simulink model "Pt_Diff_CS803"  (Simulink 7.0)
settings: Solver=ode45  StartTime=0  StopTime=20  FixedStep=TSTEP  RelTol=1e-3
PreLoadFcn:
  | cd extensions\simulink\pt_diff
  | Run_ft4wd_eclass
  | lsd_parameta_eclass
  | cd ..\..\..
undefined symbols (not defined in the file): LOCKED_FD_DAMP, LOCKED_FD_K, LOCKED_FD_OPT, LOCKED_RD_DAMP, LOCKED_RD_K, LOCKED_RD_OPT, LOCKED_XC_DAMP, LOCKED_XC_K, LOCKED_XC_OPT, M_DIFF_FD_TABLE, M_DIFF_RD_TABLE, M_DIFF_XC_TABLE, R_EFF_F_FD, R_EFF_F_RD, R_EFF_F_XC, R_EFF_R_FD, R_EFF_R_RD, R_EFF_R_XC, R_GEAR_FD, R_GEAR_RD, R_GEAR_XC, R_REAR_XC
libraries: Solver_SF x1
settings Model: Creator=dhall  LastModifiedBy=ywata  ExtModeTrigMode=oneshot  ExtModeArmWhenConnect=off
settings DataIOCC: LimitDataPoints=off  SaveOutput=off  SaveTime=off  SignalLoggingName=sigsOut
settings OptimizationCC: BooleanDataType=off
settings DebuggingCC: SaveWithParameterizedLinksMsg=none  SignalResolutionControl=TryResolveAllWithWarning  SolverPrmCheckMsg=none  MultiTaskDSMMsg=warning  MultiTaskCondExecSysMsg=none  StrictBusMsg=None
settings HardwareCC: TargetUnknown=on
settings RTWCC: IncludeERTFirstTime=on
settings GRTTargetCC: TargetFcnLib=ansi_tfl_tmw.mat  ModelReferenceCompliant=off  MatFileLogging=off

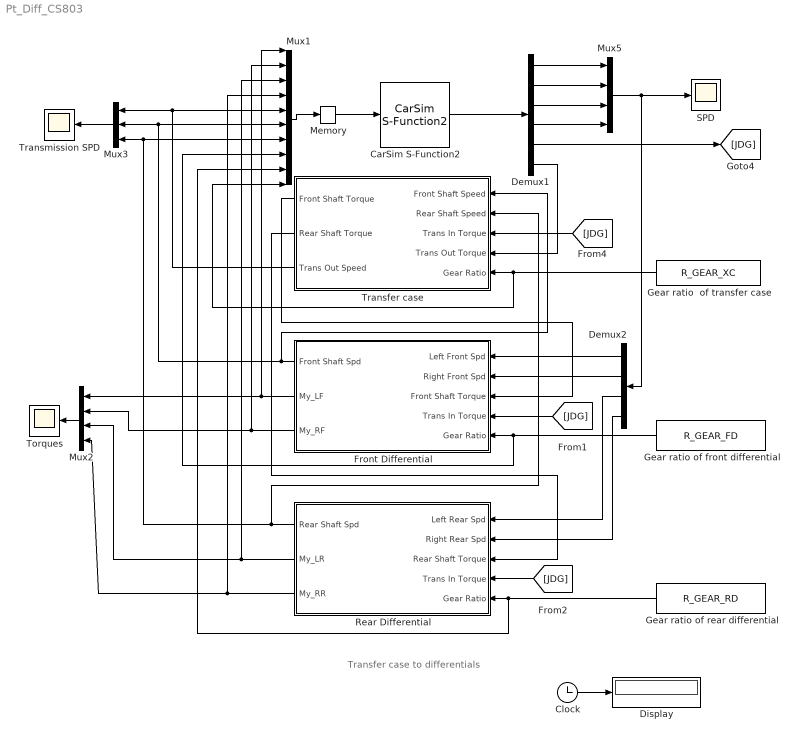
== system Pt_Diff_CS803 ==
  note: Transfer case to differentials
  CarSim S-Function2 : Solver_SF/CarSim S-Function2  Priority=1  VehicleCode=???
      settings: AttributesFormatString=Vehicle Code: %<VehicleCode>
  Clock : Clock
      settings: Decimation=10
  Demux1 : Demux  Outputs=6
  Demux2 : Demux  Orientation=left
  Display : Display
  "Front Differential " : Subsystem  Orientation=left
  Gear ratio  of transfer case : Constant  Orientation=left  Value=R_GEAR_XC  OutDataType=sfix(16)  OutScaling=2^0
  Gear ratio of front differential : Constant  Orientation=left  Value=R_GEAR_FD  OutDataType=sfix(16)  OutScaling=2^0
  Gear ratio of rear differential : Constant  Orientation=left  Value=R_GEAR_RD  OutDataType=sfix(16)  OutScaling=2^0
  Memory : Memory
  Mux1 : Mux  Inputs=10
  Mux2 : Mux  Orientation=left
  Mux3 : Mux  Orientation=left  Inputs=3
  Mux5 : Mux
  Rear Differential : Subsystem  Orientation=left
  SPD : Scope
      settings: YMin=-68.0473  YMax=1340.24
  Torques : Scope
      settings: YMin=0  YMax=1750
  Transfer case : Subsystem  Orientation=left
  Transmission SPD : Scope
      settings: YMin=-111.446  YMax=3683.73
  wires:
  Mux2/1 -> Torques/1
  "Front Differential "/1(Front Shaft Spd) -> Transfer case/1(Front Shaft Speed), Mux1/6, Mux3/2
  Rear Differential/1(Rear Shaft Spd) -> Transfer case/2(Rear Shaft Speed), Mux1/7, Mux3/3
  Transfer case/1(Front Shaft Torque) -> "Front Differential "/3(Front Shaft Torque)
  Transfer case/2(Rear Shaft Torque) -> Rear Differential/3(Rear Shaft Torque)
  [JDG] -> Rear Differential/4(Trans In Torque)
  [JDG] -> Transfer case/3(Trans In Torque)
  Mux5/1 -> SPD/1, Demux2/1
  Demux2/1 -> "Front Differential "/1(Left Front Spd)
  Demux2/2 -> "Front Differential "/2(Right Front Spd)
  Demux2/3 -> Rear Differential/1(Left Rear Spd)
  Demux2/4 -> Rear Differential/2(Right Rear Spd)
  [JDG] -> "Front Differential "/4(Trans In Torque)
  Mux1/1 -> Memory/1
  "Front Differential "/2(My_LF) -> Mux1/1, Mux2/1
  "Front Differential "/3(My_RF) -> Mux1/2, Mux2/2
  Rear Differential/2(My_LR) -> Mux1/3, Mux2/3
  Rear Differential/3(My_RR) -> Mux1/4, Mux2/4
  Gear ratio of rear differential/1 -> Rear Differential/5(Gear Ratio), Mux1/9
  Gear ratio of front differential/1 -> "Front Differential "/5(Gear Ratio), Mux1/8
  Gear ratio  of transfer case/1 -> Transfer case/5(Gear Ratio), Mux1/10
  Transfer case/3(Trans Out Speed) -> Mux1/5, Mux3/1
  Clock/1 -> Display/1
  CarSim S-Function2/1 -> Demux1/1
  Memory/1 -> CarSim S-Function2/1
  Mux3/1 -> Transmission SPD/1
  Demux1/1 -> Mux5/1
  Demux1/2 -> Mux5/2
  Demux1/3 -> Mux5/3
  Demux1/4 -> Mux5/4
  Demux1/5 -> [JDG]
  Demux1/6 -> Transfer case/4(Trans Out Torque)

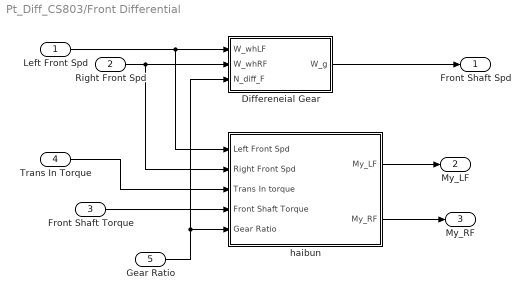
== system Pt_Diff_CS803/Front Differential  ==
  Left Front Spd : Inport  OutDataType=sfix(16)  OutScaling=2^0
  Right Front Spd : Inport  Port=2  OutDataType=sfix(16)  OutScaling=2^0
  Front Shaft Torque : Inport  Port=3  OutDataType=sfix(16)  OutScaling=2^0
  Trans In Torque : Inport  Port=4  OutDataType=sfix(16)  OutScaling=2^0
  Gear Ratio : Inport  Port=5  OutDataType=sfix(16)  OutScaling=2^0
  Differeneial Gear : Subsystem
  haibun : Subsystem
  Front Shaft Spd : Outport
  My_LF : Outport  Port=2
  My_RF : Outport  Port=3
  wires:
  haibun/2(My_RF) -> My_RF/1
  haibun/1(My_LF) -> My_LF/1
  Right Front Spd/1 -> Differeneial Gear/2(W_whRF), haibun/2(Right Front Spd)
  Left Front Spd/1 -> Differeneial Gear/1(W_whLF), haibun/1(Left Front Spd)
  Gear Ratio/1 -> haibun/5(Gear Ratio), Differeneial Gear/3(N_diff_F)
  Differeneial Gear/1(W_g) -> Front Shaft Spd/1
  Front Shaft Torque/1 -> haibun/4(Front Shaft Torque)
  Trans In Torque/1 -> haibun/3(Trans In torque)

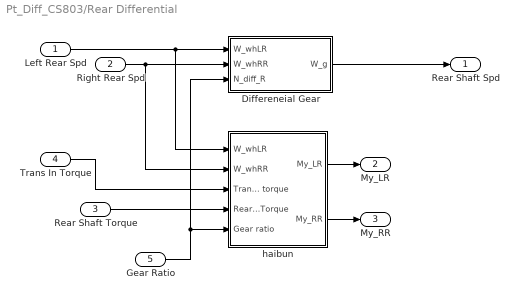
== system Pt_Diff_CS803/Rear Differential ==
  Left Rear Spd : Inport  OutDataType=sfix(16)  OutScaling=2^0
  Right Rear Spd : Inport  Port=2  OutDataType=sfix(16)  OutScaling=2^0
  Rear Shaft Torque : Inport  Port=3  OutDataType=sfix(16)  OutScaling=2^0
  Trans In Torque : Inport  Port=4  OutDataType=sfix(16)  OutScaling=2^0
  Gear Ratio : Inport  Port=5  OutDataType=sfix(16)  OutScaling=2^0
  Differeneial Gear : Subsystem
  haibun : Subsystem
  Rear Shaft Spd : Outport
  My_LR : Outport  Port=2
  My_RR : Outport  Port=3
  wires:
  Trans In Torque/1 -> haibun/3(Trans In torque)
  Rear Shaft Torque/1 -> haibun/4(Rear Shaft Torque)
  Differeneial Gear/1(W_g) -> Rear Shaft Spd/1
  Gear Ratio/1 -> Differeneial Gear/3(N_diff_R), haibun/5(Gear ratio)
  Left Rear Spd/1 -> haibun/1(W_whLR), Differeneial Gear/1(W_whLR)
  Right Rear Spd/1 -> haibun/2(W_whRR), Differeneial Gear/2(W_whRR)
  haibun/1(My_LR) -> My_LR/1
  haibun/2(My_RR) -> My_RR/1

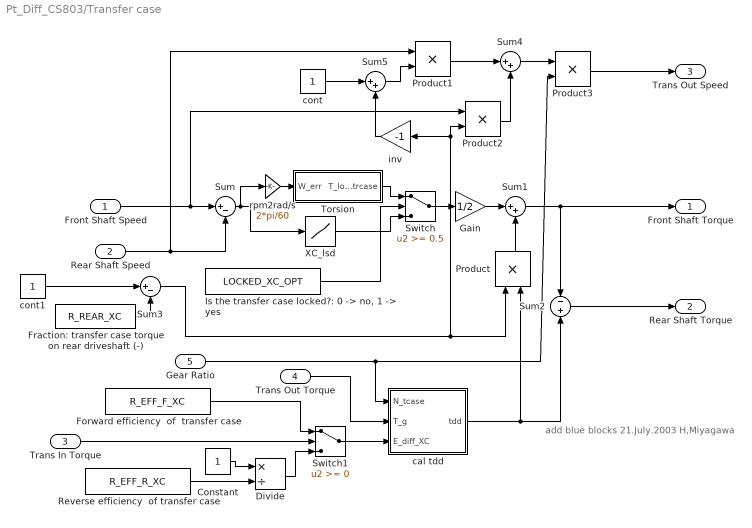
== system Pt_Diff_CS803/Transfer case ==
  note: add blue blocks
      | 21.July.2003
      | H,Miyagawa
  Front Shaft Speed : Inport  OutDataType=sfix(16)  OutScaling=2^0
  Rear Shaft Speed : Inport  Port=2  OutDataType=sfix(16)  OutScaling=2^0
  Trans In Torque : Inport  Port=3  OutDataType=sfix(16)  OutScaling=2^0
  Trans Out Torque : Inport  Port=4  OutDataType=sfix(16)  OutScaling=2^0
  Gear Ratio : Inport  Port=5  OutDataType=sfix(16)  OutScaling=2^0
  Constant : Constant  OutDataType=sfix(16)  OutScaling=2^0
  Divide : Product  Inputs=*/  OutDataType=sfix(16)  OutScaling=2^0  InputSameDT=on
  Forward efficiency  of  transfer case : Constant  Value=R_EFF_F_XC  OutDataType=sfix(16)  OutScaling=2^0
  Fraction: transfer case torque on rear driveshaft (-) : Constant  Value=R_REAR_XC  OutDataType=sfix(16)  OutScaling=2^0
  Gain : Gain  Gain=1/2  ParameterDataType=sfix(16)  ParameterScaling=2^0  OutDataType=sfix(16)  OutScaling=2^0  SaturateOnIntegerOverflow=on
  "Is the transfer case locked?: 0 -> no, 1 -> yes" : Constant  Value=LOCKED_XC_OPT  OutDataType=sfix(16)  OutScaling=2^0
  Product : Product  Orientation=up  OutDataType=sfix(16)  OutScaling=2^0  SaturateOnIntegerOverflow=on  InputSameDT=on
  Product1 : Product  OutDataType=sfix(16)  OutScaling=2^0  SaturateOnIntegerOverflow=on  InputSameDT=on
  Product2 : Product  OutDataType=sfix(16)  OutScaling=2^0  SaturateOnIntegerOverflow=on  InputSameDT=on
  Product3 : Product  OutDataType=sfix(16)  OutScaling=2^0  SaturateOnIntegerOverflow=on  InputSameDT=on
  Reverse efficiency  of transfer case : Constant  Value=R_EFF_R_XC  OutDataType=sfix(16)  OutScaling=2^0
  Sum : Sum  Inputs=|+-  OutDataType=sfix(16)  OutScaling=2^0  SaturateOnIntegerOverflow=on  InputSameDT=on
  Sum1 : Sum  Inputs=|++  OutDataType=sfix(16)  OutScaling=2^0  SaturateOnIntegerOverflow=on  InputSameDT=on
  Sum2 : Sum  Inputs=-|+  OutDataType=sfix(16)  OutScaling=2^0  SaturateOnIntegerOverflow=on  InputSameDT=on
  Sum3 : Sum  Inputs=|+-  OutDataType=sfix(16)  OutScaling=2^0  SaturateOnIntegerOverflow=on  InputSameDT=on
  Sum4 : Sum  Inputs=|++  OutDataType=sfix(16)  OutScaling=2^0  SaturateOnIntegerOverflow=on  InputSameDT=on
  Sum5 : Sum  Inputs=|++  OutDataType=sfix(16)  OutScaling=2^0  SaturateOnIntegerOverflow=on  InputSameDT=on
  Switch : Switch  Threshold=0.5  SaturateOnIntegerOverflow=on  InputSameDT=on
  Switch1 : Switch  SaturateOnIntegerOverflow=on  InputSameDT=on
  Torsion : Subsystem
  XC_lsd : Lookup  InputValues=M_DIFF_XC_TABLE(:,1)  Table=M_DIFF_XC_TABLE(:,2)  OutDataType=sfix(16)  OutScaling=2^0  SaturateOnIntegerOverflow=on
  cal tdd : Subsystem
  cont : Constant  OutDataType=sfix(16)  OutScaling=2^0
  cont1 : Constant  OutDataType=sfix(16)  OutScaling=2^0
  inv : Gain  Orientation=left  Gain=-1  ParameterDataType=sfix(16)  ParameterScaling=2^0  OutDataType=sfix(16)  OutScaling=2^0  SaturateOnIntegerOverflow=on
  rpm2rad/s : Gain  Gain=2*pi/60  ParameterDataType=sfix(16)  ParameterScaling=2^0  OutDataType=sfix(16)  OutScaling=2^0  SaturateOnIntegerOverflow=on
  Front Shaft Torque : Outport
  Rear Shaft Torque : Outport  Port=2
  Trans Out Speed : Outport  Port=3
  wires:
  Sum1/1 -> Sum2/1, Front Shaft Torque/1
  Sum2/1 -> Rear Shaft Torque/1
  cal tdd/1(tdd) -> Product/2, Sum2/2
  Switch1/1 -> cal tdd/3(E_diff_XC)
  Forward efficiency  of  transfer case/1 -> Switch1/1
  Trans In Torque/1 -> Switch1/2
  Trans Out Torque/1 -> cal tdd/2(T_g)
  Product/1 -> Sum1/2
  Gain/1 -> Sum1/1
  Switch/1 -> Gain/1
  XC_lsd/1 -> Switch/3
  "Is the transfer case locked?: 0 -> no, 1 -> yes"/1 -> Switch/2
  Sum/1 -> XC_lsd/1, rpm2rad/s/1
  Torsion/1(T_lock_trcase) -> Switch/1
  Product2/1 -> Sum4/2
  Product1/1 -> Sum4/1
  Sum4/1 -> Product3/1
  Product3/1 -> Trans Out Speed/1
  Gear Ratio/1 -> cal tdd/1(N_tcase), Product3/2
  Sum5/1 -> Product1/2
  cont/1 -> Sum5/1
  inv/1 -> Sum5/2
  Front Shaft Speed/1 -> Sum/1, Product2/1
  Rear Shaft Speed/1 -> Sum/2, Product1/1
  Fraction: transfer case torque on rear driveshaft (-)/1 -> Sum3/2
  Sum3/1 -> Product/1, Product2/2, inv/1
  cont1/1 -> Sum3/1
  Constant/1 -> Divide/1
  Reverse efficiency  of transfer case/1 -> Divide/2
  Divide/1 -> Switch1/3
  rpm2rad/s/1 -> Torsion/1(W_err)

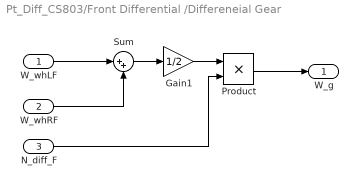
== system Pt_Diff_CS803/Front Differential /Differeneial Gear ==
  W_whLF : Inport  OutDataType=sfix(16)  OutScaling=2^0
  W_whRF : Inport  Port=2  OutDataType=sfix(16)  OutScaling=2^0
  N_diff_F : Inport  Port=3  OutDataType=sfix(16)  OutScaling=2^0
  Gain1 : Gain  Gain=1/2  ParameterDataType=sfix(16)  ParameterScaling=2^0  OutDataType=sfix(16)  OutScaling=2^0  SaturateOnIntegerOverflow=on
  Product : Product  OutDataType=sfix(16)  OutScaling=2^0  SaturateOnIntegerOverflow=on  InputSameDT=on
  Sum : Sum  Inputs=|++  OutDataType=sfix(16)  OutScaling=2^0  SaturateOnIntegerOverflow=on  InputSameDT=on
  W_g : Outport
  wires:
  Product/1 -> W_g/1
  Gain1/1 -> Product/1
  W_whRF/1 -> Sum/2
  W_whLF/1 -> Sum/1
  N_diff_F/1 -> Product/2
  Sum/1 -> Gain1/1

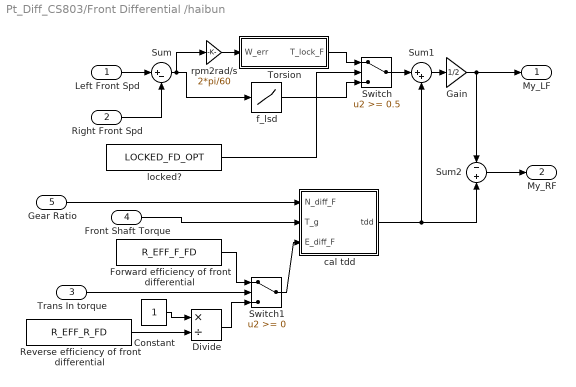
== system Pt_Diff_CS803/Front Differential /haibun ==
  Left Front Spd : Inport  OutDataType=sfix(16)  OutScaling=2^0
  Right Front Spd : Inport  Port=2  OutDataType=sfix(16)  OutScaling=2^0
  Trans In torque : Inport  Port=3  OutDataType=sfix(16)  OutScaling=2^0
  Front Shaft Torque : Inport  Port=4  OutDataType=sfix(16)  OutScaling=2^0
  Gear Ratio : Inport  Port=5  OutDataType=sfix(16)  OutScaling=2^0
  Constant : Constant  OutDataType=sfix(16)  OutScaling=2^0
  Divide : Product  Inputs=*/  OutDataType=sfix(16)  OutScaling=2^0  InputSameDT=on
  Forward efficiency of front differential : Constant  Value=R_EFF_F_FD  OutDataType=sfix(16)  OutScaling=2^0
  Gain : Gain  Gain=1/2  ParameterDataType=sfix(16)  ParameterScaling=2^0  OutDataType=sfix(16)  OutScaling=2^0  SaturateOnIntegerOverflow=on
  Reverse efficiency of front differential : Constant  Value=R_EFF_R_FD  OutDataType=sfix(16)  OutScaling=2^0
  Sum : Sum  Inputs=|+-  OutDataType=sfix(16)  OutScaling=2^0  SaturateOnIntegerOverflow=on  InputSameDT=on
  Sum1 : Sum  Inputs=|++  OutDataType=sfix(16)  OutScaling=2^0  SaturateOnIntegerOverflow=on  InputSameDT=on
  Sum2 : Sum  Inputs=-|+  OutDataType=sfix(16)  OutScaling=2^0  SaturateOnIntegerOverflow=on  InputSameDT=on
  Switch : Switch  Threshold=0.5  SaturateOnIntegerOverflow=on  InputSameDT=on
  Switch1 : Switch  SaturateOnIntegerOverflow=on  InputSameDT=on
  Torsion : Subsystem
  cal tdd : Subsystem
  f_lsd : Lookup  InputValues=M_DIFF_FD_TABLE(:,1)  Table=M_DIFF_FD_TABLE(:,2)  OutDataType=sfix(16)  OutScaling=2^0  SaturateOnIntegerOverflow=on
  locked? : Constant  Value=LOCKED_FD_OPT  OutDataType=sfix(16)  OutScaling=2^0
  rpm2rad/s : Gain  Gain=2*pi/60  ParameterDataType=sfix(16)  ParameterScaling=2^0  OutDataType=sfix(16)  OutScaling=2^0  SaturateOnIntegerOverflow=on
  My_LF : Outport
  My_RF : Outport  Port=2
  wires:
  Front Shaft Torque/1 -> cal tdd/2(T_g)
  Trans In torque/1 -> Switch1/2
  Forward efficiency of front differential/1 -> Switch1/1
  Switch1/1 -> cal tdd/3(E_diff_F)
  Left Front Spd/1 -> Sum/1
  Right Front Spd/1 -> Sum/2
  cal tdd/1(tdd) -> Sum1/2, Sum2/2
  Sum2/1 -> My_RF/1
  Gear Ratio/1 -> cal tdd/1(N_diff_F)
  Torsion/1(T_lock_F) -> Switch/1
  Switch/1 -> Sum1/1
  Sum1/1 -> Gain/1
  Gain/1 -> My_LF/1, Sum2/1
  Sum/1 -> f_lsd/1, rpm2rad/s/1
  locked?/1 -> Switch/2
  f_lsd/1 -> Switch/3
  Constant/1 -> Divide/1
  Reverse efficiency of front differential/1 -> Divide/2
  Divide/1 -> Switch1/3
  rpm2rad/s/1 -> Torsion/1(W_err)

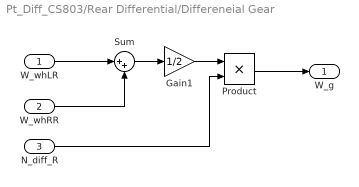
== system Pt_Diff_CS803/Rear Differential/Differeneial Gear ==
  W_whLR : Inport  OutDataType=sfix(16)  OutScaling=2^0
  W_whRR : Inport  Port=2  OutDataType=sfix(16)  OutScaling=2^0
  N_diff_R : Inport  Port=3  OutDataType=sfix(16)  OutScaling=2^0
  Gain1 : Gain  Gain=1/2  ParameterDataType=sfix(16)  ParameterScaling=2^0  OutDataType=sfix(16)  OutScaling=2^0  SaturateOnIntegerOverflow=on
  Product : Product  OutDataType=sfix(16)  OutScaling=2^0  SaturateOnIntegerOverflow=on  InputSameDT=on
  Sum : Sum  Inputs=|++  OutDataType=sfix(16)  OutScaling=2^0  SaturateOnIntegerOverflow=on  InputSameDT=on
  W_g : Outport
  wires:
  Sum/1 -> Gain1/1
  N_diff_R/1 -> Product/2
  W_whLR/1 -> Sum/1
  W_whRR/1 -> Sum/2
  Gain1/1 -> Product/1
  Product/1 -> W_g/1

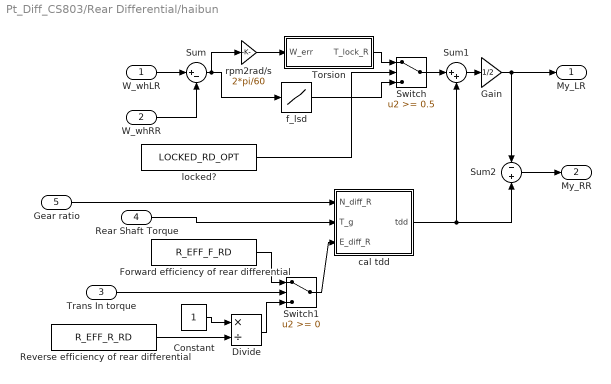
== system Pt_Diff_CS803/Rear Differential/haibun ==
  W_whLR : Inport  OutDataType=sfix(16)  OutScaling=2^0
  W_whRR : Inport  Port=2  OutDataType=sfix(16)  OutScaling=2^0
  Trans In torque : Inport  Port=3  OutDataType=sfix(16)  OutScaling=2^0
  Rear Shaft Torque : Inport  Port=4  OutDataType=sfix(16)  OutScaling=2^0
  Gear ratio : Inport  Port=5  OutDataType=sfix(16)  OutScaling=2^0
  Constant : Constant  OutDataType=sfix(16)  OutScaling=2^0
  Divide : Product  Inputs=*/  OutDataType=sfix(16)  OutScaling=2^0  InputSameDT=on
  Forward efficiency of rear differential : Constant  Value=R_EFF_F_RD  OutDataType=sfix(16)  OutScaling=2^0
  Gain : Gain  Gain=1/2  ParameterDataType=sfix(16)  ParameterScaling=2^0  OutDataType=sfix(16)  OutScaling=2^0  SaturateOnIntegerOverflow=on
  Reverse efficiency of rear differential : Constant  Value=R_EFF_R_RD  OutDataType=sfix(16)  OutScaling=2^0
  Sum : Sum  Inputs=|+-  OutDataType=sfix(16)  OutScaling=2^0  SaturateOnIntegerOverflow=on  InputSameDT=on
  Sum1 : Sum  Inputs=|++  OutDataType=sfix(16)  OutScaling=2^0  SaturateOnIntegerOverflow=on  InputSameDT=on
  Sum2 : Sum  Inputs=-|+  OutDataType=sfix(16)  OutScaling=2^0  SaturateOnIntegerOverflow=on  InputSameDT=on
  Switch : Switch  Threshold=0.5  SaturateOnIntegerOverflow=on  InputSameDT=on
  Switch1 : Switch  SaturateOnIntegerOverflow=on  InputSameDT=on
  Torsion : Subsystem
  cal tdd : Subsystem
  f_lsd : Lookup  InputValues=M_DIFF_RD_TABLE(:,1)  Table=M_DIFF_RD_TABLE(:,2)  OutDataType=sfix(16)  OutScaling=2^0  SaturateOnIntegerOverflow=on
  locked? : Constant  Value=LOCKED_RD_OPT  OutDataType=sfix(16)  OutScaling=2^0
  rpm2rad/s : Gain  Gain=2*pi/60  ParameterDataType=sfix(16)  ParameterScaling=2^0  OutDataType=sfix(16)  OutScaling=2^0  SaturateOnIntegerOverflow=on
  My_LR : Outport
  My_RR : Outport  Port=2
  wires:
  f_lsd/1 -> Switch/3
  locked?/1 -> Switch/2
  Sum/1 -> f_lsd/1, rpm2rad/s/1
  Gain/1 -> Sum2/1, My_LR/1
  Sum1/1 -> Gain/1
  Switch/1 -> Sum1/1
  Torsion/1(T_lock_R) -> Switch/1
  Gear ratio/1 -> cal tdd/1(N_diff_R)
  Sum2/1 -> My_RR/1
  cal tdd/1(tdd) -> Sum2/2, Sum1/2
  W_whRR/1 -> Sum/2
  W_whLR/1 -> Sum/1
  Switch1/1 -> cal tdd/3(E_diff_R)
  Forward efficiency of rear differential/1 -> Switch1/1
  Trans In torque/1 -> Switch1/2
  Rear Shaft Torque/1 -> cal tdd/2(T_g)
  Constant/1 -> Divide/1
  Reverse efficiency of rear differential/1 -> Divide/2
  Divide/1 -> Switch1/3
  rpm2rad/s/1 -> Torsion/1(W_err)

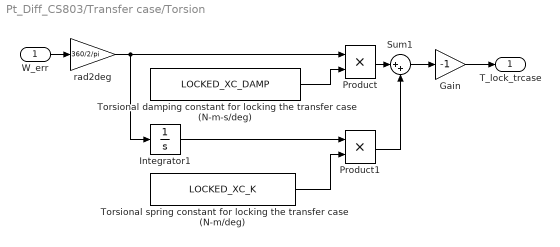
== system Pt_Diff_CS803/Transfer case/Torsion ==
  W_err : Inport  OutDataType=sfix(16)  OutScaling=2^0
  Gain : Gain  Gain=-1  ParameterDataType=sfix(16)  ParameterScaling=2^0  OutDataType=sfix(16)  OutScaling=2^0  SaturateOnIntegerOverflow=on
  Integrator1 : Integrator
  Product : Product  OutDataType=sfix(16)  OutScaling=2^0  SaturateOnIntegerOverflow=on  InputSameDT=on
  Product1 : Product  OutDataType=sfix(16)  OutScaling=2^0  SaturateOnIntegerOverflow=on  InputSameDT=on
  Sum1 : Sum  Inputs=|++  OutDataType=sfix(16)  OutScaling=2^0  SaturateOnIntegerOverflow=on  InputSameDT=on
  Torsional damping constant for locking the transfer case (N-m-s/deg) : Constant  Value=LOCKED_XC_DAMP  OutDataType=sfix(16)  OutScaling=2^0
  Torsional spring constant for locking the transfer case (N-m/deg) : Constant  Value=LOCKED_XC_K  OutDataType=sfix(16)  OutScaling=2^0
  rad2deg : Gain  Gain=360/2/pi  ParameterDataType=sfix(16)  ParameterScaling=2^0  OutDataType=sfix(16)  OutScaling=2^0  SaturateOnIntegerOverflow=on
  T_lock_trcase : Outport
  wires:
  Torsional spring constant for locking the transfer case (N-m/deg)/1 -> Product1/2
  Integrator1/1 -> Product1/1
  Torsional damping constant for locking the transfer case (N-m-s/deg)/1 -> Product/2
  Product/1 -> Sum1/1
  Product1/1 -> Sum1/2
  Sum1/1 -> Gain/1
  Gain/1 -> T_lock_trcase/1
  W_err/1 -> rad2deg/1
  rad2deg/1 -> Product/1, Integrator1/1

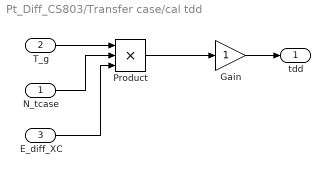
== system Pt_Diff_CS803/Transfer case/cal tdd ==
  N_tcase : Inport  OutDataType=sfix(16)  OutScaling=2^0
  T_g : Inport  Port=2  OutDataType=sfix(16)  OutScaling=2^0
  E_diff_XC : Inport  Port=3  OutDataType=sfix(16)  OutScaling=2^0
  Gain : Gain  ParameterDataType=sfix(16)  ParameterScaling=2^0  OutDataType=sfix(16)  OutScaling=2^0  SaturateOnIntegerOverflow=on
  Product : Product  Inputs=3  OutDataType=sfix(16)  OutScaling=2^0  SaturateOnIntegerOverflow=on  InputSameDT=on
  tdd : Outport
  wires:
  T_g/1 -> Product/1
  N_tcase/1 -> Product/2
  E_diff_XC/1 -> Product/3
  Product/1 -> Gain/1
  Gain/1 -> tdd/1

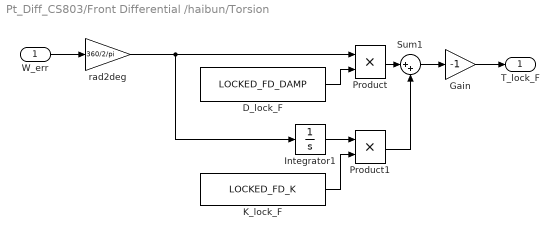
== system Pt_Diff_CS803/Front Differential /haibun/Torsion ==
  W_err : Inport  OutDataType=sfix(16)  OutScaling=2^0
  D_lock_F : Constant  Value=LOCKED_FD_DAMP  OutDataType=sfix(16)  OutScaling=2^0
  Gain : Gain  Gain=-1  ParameterDataType=sfix(16)  ParameterScaling=2^0  OutDataType=sfix(16)  OutScaling=2^0  SaturateOnIntegerOverflow=on
  Integrator1 : Integrator
  K_lock_F : Constant  Value=LOCKED_FD_K  OutDataType=sfix(16)  OutScaling=2^0
  Product : Product  OutDataType=sfix(16)  OutScaling=2^0  SaturateOnIntegerOverflow=on  InputSameDT=on
  Product1 : Product  OutDataType=sfix(16)  OutScaling=2^0  SaturateOnIntegerOverflow=on  InputSameDT=on
  Sum1 : Sum  Inputs=|++  OutDataType=sfix(16)  OutScaling=2^0  SaturateOnIntegerOverflow=on  InputSameDT=on
  rad2deg : Gain  Gain=360/2/pi  ParameterDataType=sfix(16)  ParameterScaling=2^0  OutDataType=sfix(16)  OutScaling=2^0  SaturateOnIntegerOverflow=on
  T_lock_F : Outport
  wires:
  rad2deg/1 -> Integrator1/1, Product/1
  W_err/1 -> rad2deg/1
  Gain/1 -> T_lock_F/1
  Sum1/1 -> Gain/1
  D_lock_F/1 -> Product/2
  Integrator1/1 -> Product1/1
  K_lock_F/1 -> Product1/2
  Product1/1 -> Sum1/2
  Product/1 -> Sum1/1

== system Pt_Diff_CS803/Front Differential /haibun/cal tdd ==
  N_diff_F : Inport  OutDataType=sfix(16)  OutScaling=2^0
  T_g : Inport  Port=2  OutDataType=sfix(16)  OutScaling=2^0
  E_diff_F : Inport  Port=3  OutDataType=sfix(16)  OutScaling=2^0
  Gain : Gain  ParameterDataType=sfix(16)  ParameterScaling=2^0  OutDataType=sfix(16)  OutScaling=2^0  SaturateOnIntegerOverflow=on
  Product : Product  Inputs=3  OutDataType=sfix(16)  OutScaling=2^0  SaturateOnIntegerOverflow=on  InputSameDT=on
  tdd : Outport
  wires:
  Gain/1 -> tdd/1
  Product/1 -> Gain/1
  E_diff_F/1 -> Product/3
  N_diff_F/1 -> Product/2
  T_g/1 -> Product/1

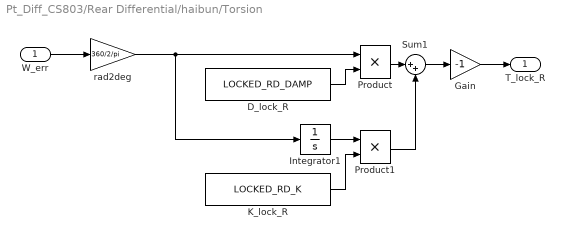
== system Pt_Diff_CS803/Rear Differential/haibun/Torsion ==
  W_err : Inport  OutDataType=sfix(16)  OutScaling=2^0
  D_lock_R : Constant  Value=LOCKED_RD_DAMP  OutDataType=sfix(16)  OutScaling=2^0
  Gain : Gain  Gain=-1  ParameterDataType=sfix(16)  ParameterScaling=2^0  OutDataType=sfix(16)  OutScaling=2^0  SaturateOnIntegerOverflow=on
  Integrator1 : Integrator
  K_lock_R : Constant  Value=LOCKED_RD_K  OutDataType=sfix(16)  OutScaling=2^0
  Product : Product  OutDataType=sfix(16)  OutScaling=2^0  SaturateOnIntegerOverflow=on  InputSameDT=on
  Product1 : Product  OutDataType=sfix(16)  OutScaling=2^0  SaturateOnIntegerOverflow=on  InputSameDT=on
  Sum1 : Sum  Inputs=|++  OutDataType=sfix(16)  OutScaling=2^0  SaturateOnIntegerOverflow=on  InputSameDT=on
  rad2deg : Gain  Gain=360/2/pi  ParameterDataType=sfix(16)  ParameterScaling=2^0  OutDataType=sfix(16)  OutScaling=2^0  SaturateOnIntegerOverflow=on
  T_lock_R : Outport
  wires:
  rad2deg/1 -> Integrator1/1, Product/1
  W_err/1 -> rad2deg/1
  Product/1 -> Sum1/1
  Product1/1 -> Sum1/2
  K_lock_R/1 -> Product1/2
  Integrator1/1 -> Product1/1
  D_lock_R/1 -> Product/2
  Sum1/1 -> Gain/1
  Gain/1 -> T_lock_R/1

== system Pt_Diff_CS803/Rear Differential/haibun/cal tdd ==
  N_diff_R : Inport  OutDataType=sfix(16)  OutScaling=2^0
  T_g : Inport  Port=2  OutDataType=sfix(16)  OutScaling=2^0
  E_diff_R : Inport  Port=3  OutDataType=sfix(16)  OutScaling=2^0
  Gain : Gain  ParameterDataType=sfix(16)  ParameterScaling=2^0  OutDataType=sfix(16)  OutScaling=2^0  SaturateOnIntegerOverflow=on
  Product : Product  Inputs=3  OutDataType=sfix(16)  OutScaling=2^0  SaturateOnIntegerOverflow=on  InputSameDT=on
  tdd : Outport
  wires:
  T_g/1 -> Product/1
  N_diff_R/1 -> Product/2
  E_diff_R/1 -> Product/3
  Product/1 -> Gain/1
  Gain/1 -> tdd/1
